simulink model "eCS_Algo_Simulation_2015b_opti - Copy"  (R2015b)
settings: Solver=ode1  StartTime=0.0  StopTime=3  FixedStep=1/80000  RelTol=1e-3
PreLoadFcn:
  | if exist('tl_preloadfcn','file'), tl_preloadfcn(gcs,402); end
PostLoadFcn:
  | , if any(exist('dsrtsu_mdlpostloadfcn', 'file') == [2, 3, 6]), try dsrtsu_mdlpostloadfcn('Execute', bdroot); catch fprintf('Error in PostLoadFcn (dsrtsu_mdlpostloadfcn) for model "%s":\n %s\n', bdroot, lasterr); end, end,
  | if exist('tl_postloadfcn','file'), tl_postloadfcn(gcs,402); end
InitFcn:
  | Omegan=1.3024e+03;
  | xi=0.9; %0.48
  | K=0.1931;
  | K1=0.0198;
  | TauLocked=0.00255;
  | TauUnLocked=0.0042;
  | Kp=1/(2*K1);
  | Ki=Kp/((TauLocked+TauUnLocked)/2);
  | if exist('tlds_init','file'), tlds_init(gcs); end
StartFcn:
  | if exist('tlds_start','file'), tlds_start(gcs); end
StopFcn:
  | if exist('tlds_stop','file'), tlds_stop(gcs); end
model workspace (MAT data in the model file):
  au8PrevExecProfile = [0 0 0 0 0 0]
values from neighbouring files (symbols this model uses):
  AccSensor = 5    [Parameter_eCS_Algo.m]
  AlgoType = 0    [Parameter_eCS_Algo.m]
  Cxy = 1*0.017    (= 0.017)    [Acc_Init_SelV1.m]
  Cxz = 1*0.017    (= 0.017)    [Acc_Init_SelV1.m]
  Cyx = 1*0.017    (= 0.017)    [Acc_Init_SelV1.m]
  Cyz = 1*0.017    (= 0.017)    [Acc_Init_SelV1.m]
  Czx = 1*0.017    (= 0.017)    [Acc_Init_SelV1.m]
  Czy = 1*0.017    (= 0.017)    [Acc_Init_SelV1.m]
  Forced_Oscillation = 0    [Parameter_eCS_Algo.m]    (also in run_Rotation_sim.m = run)
  FreqTemperature = 10    [Acc_Init_SelV1.m]
  MaxSensorOffset = 0.3    [Acc_Init_SelV1.m]
  Mean_x_noise = 4e-3    (= 0.004)    [Acc_Init_SelV1.m]
  Mean_y_noise = 4e-3    (= 0.004)    [Acc_Init_SelV1.m]
  Mean_z_noise = 4e-3    (= 0.004)    [Acc_Init_SelV1.m]
  ODR = 8000    [Acc_Init_SelV1.m]
  offsetcorrection_on_off = 0    [Parameter_eCS_Algo.m]
  phi_pulse_rotation = 0    [Parameter_eCS_Algo.m]    (also in run_Rotation_sim.m = angle)
  pulsetype = 2    [Parameter_eCS_Algo.m]    (also in run_simulation.m = j; run_simulation_ActiveX.m = j)
  Range = 4    [Acc_Init_SelV1.m]
  sensitivity_optimisation = 0    [Parameter_eCS_Algo.m]
  TempBias = 0    [Acc_Init_SelV1.m]
  TemperatureAmp = 0    [Acc_Init_SelV1.m]
  Var_x_noise = 1.84e-9    (= 1.84e-09)    [Acc_Init_SelV1.m]
  Var_y_noise = 2.025e-09    [Acc_Init_SelV1.m]
  Var_z_noise = 1.374e-09    [Acc_Init_SelV1.m]
  w_x = 2*pi*F_x    (= 376.991118431)    [Acc_Init_SelV1.m]
  w_y = 2*pi*F_y    (= 376.991118431)    [Acc_Init_SelV1.m]
  w_z = 2*pi*F_z    (= 376.991118431)    [Acc_Init_SelV1.m]
  x_max_temp_drift = 0.061    [Acc_Init_SelV1.m]
  x_offset_enable = 0    [Acc_Init_SelV1.m]
  x_run_to_run_drift = 0.0    (= 0)    [Acc_Init_SelV1.m]
  x_temp_co_drift = 0.000    (= 0)    [Acc_Init_SelV1.m]
  Xi_x = 0.7    [Acc_Init_SelV1.m]
  Xi_y = 0.7    [Acc_Init_SelV1.m]
  Xi_z = 0.7    [Acc_Init_SelV1.m]
  y_max_temp_drift = 0.061    [Acc_Init_SelV1.m]
  y_offset_enable = 0    [Acc_Init_SelV1.m]
  y_run_to_run_drift = 0.0    (= 0)    [Acc_Init_SelV1.m]
  y_temp_co_drift = 0.000    (= 0)    [Acc_Init_SelV1.m]
  z_max_temp_drift = 0.13    [Acc_Init_SelV1.m]
  z_offset_enable = 0    [Acc_Init_SelV1.m]
  z_run_to_run_drift = 0.0    (= 0)    [Acc_Init_SelV1.m]
  z_temp_co_drift = 0.000    (= 0)    [Acc_Init_SelV1.m]
undefined symbols (not defined in the file or in its folder): ddv, DiscIntNeverNeededParam, gmw_roada_x__m_s__, gmw_roada_y__m_s__, gmw_roadtime_2kHz, KSF_50_a_x, KSF_50_a_y, KSF_50_time, KSG_30_a_x, KSG_30_a_y, KSG_30_time, Meldorf_HindenburgstraAcceleration_x__m_s_2_, Meldorf_HindenburgstraAcceleration_y__m_s_2_, Meldorf_HindenburgstraAcceleration_z__m_s_2_, Meldorf_HindenburgstraTime__s_, pulse_FF27, pulse_MPDB, pulse_ODB40, pulse_ODB64, pulse_USNCAP, pulsetime_FF27, pulsetime_MPDB, pulsetime_ODB40, pulsetime_ODB64, pulsetime_USNCAP, Rauasphalt_60_a_x, Rauasphalt_60_a_y, Rauasphalt_60_time, sigbuilder_block, VW_416_2kHza_x_2kHz, VW_416_2kHza_y_2kHz, VW_416_2kHztime_2kHz
libraries: tllib x22, simulink x20, tl_autosar_lib x10, simulink_extras x7, LIB_TF_G_12_StepControl x2, LIB_TF_G_111 x1, LIB_TF_G_112 x1
(part 2 of 9)

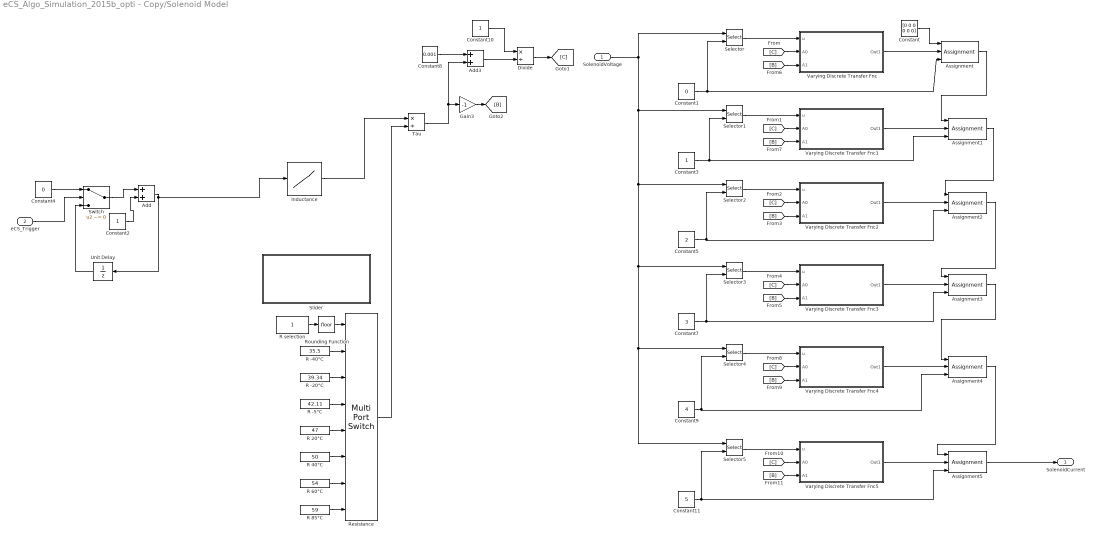
== system eCS_Algo_Simulation_2015b_opti - Copy/Solenoid Model ==
  SolenoidVoltage : Inport
  eCS_Trigger : Inport  Port=2  SampleTime=0.001
  Add : Sum
  Add3 : Sum
  Assignment{,1..5} (6 alike) : Assignment  IndexMode=Zero-based  IndexOptions=Index vector (port)  Indices=1  OutputSizes=1
  Constant : Constant  Value=[0 0 0 0 0 0]
  Constant1 : Constant  Value=0
  Constant10 : Constant
  Constant11 : Constant  Value=5
  Constant2 : Constant
  Constant3 : Constant
  Constant4 : Constant  Value=0
  Constant5 : Constant  Value=2
  Constant7 : Constant  Value=3
  Constant8 : Constant  Value=0.001
  Constant9 : Constant  Value=4
  Divide : Product  Inputs=*/
  Gain3 : Gain  Gain=-1
  Inductance : Lookup_n-D  NumberOfTableDimensions=1  BreakpointsForDimension1=[0 5 10 15 20 25 25.001]  Table=[0.262 0.2108 0.1697 0.1449 0.1286 0.1185 0.1185]  InternalRulePriority=Speed  RndMeth=Simplest  InputSameDT=on
  R -20°C : Constant  Value=39.34
  R -40°C : Constant  Value=35.5
  R -5°C : Constant  Value=42.11
  R 20°C : Constant  Value=47
  R 40°C : Constant  Value=50
  R 60°C : Constant  Value=54
  R 85°C : Constant  Value=59
  R selection : Constant
  Resistance : MultiPortSwitch  Inputs=7
  Rounding Function : Rounding
  Selector{,1..5} (6 alike) : Selector  IndexMode=Zero-based  InputPortWidth=6  IndexOptions=Index vector (port)  Indices=[1 3]  OutputSizes=1
  Slider : Subsystem  DialogController=hmiCreateDDGDialog  IsWebBlock=on  mask(MWDashboardBlock){webBlockId=75143694-038a-4636-9846-8391abf771a2, webBlockType=slider, ShowInLibBrowser=on, ShowInitialText=on, HMISrcModelName=eCS_Algo_Simulation_2015b_opti}
      mask prompts: webBlockId "WebBlock Id"; webBlockType "WebBlock Type"; HMISrcModelName "Source Model"
      mask Help: helpview([docroot '/mapfiles/simulink.map'], 'hmi_slider')
      mask Display:
      | if strcmp(get_param(bdroot(gcb),'BlockDiagramType'), 'library')
      |     image([(matlabroot) '/toolbox/simulink/hmi/icons/Slider.png']);
      | end
  Switch : Switch  Criteria=u2 ~= 0
  Tau : Product  Inputs=*/
  Unit Delay : UnitDelay  SampleTime=-1
  Varying Discrete Transfer Fnc : Subsystem
  Varying Discrete Transfer Fnc1 : Subsystem
  Varying Discrete Transfer Fnc2 : Subsystem
  Varying Discrete Transfer Fnc3 : Subsystem
  Varying Discrete Transfer Fnc4 : Subsystem
  Varying Discrete Transfer Fnc5 : Subsystem
  SolenoidCurrent : Outport
  wires:
  Constant1/1 -> Assignment/3, Selector/2
  Constant/1 -> Assignment/1
  Constant3/1 -> Assignment1/3, Selector1/2
  Assignment/1 -> Assignment1/1
  Constant2/1 -> Add/2
  Add/1 -> Unit Delay/1, Inductance/1
  Switch/1 -> Add/1
  Unit Delay/1 -> Switch/3
  Constant4/1 -> Switch/1
  eCS_Trigger/1 -> Switch/2
  Constant5/1 -> Assignment2/3, Selector2/2
  Assignment1/1 -> Assignment2/1
  Constant7/1 -> Assignment3/3, Selector3/2
  Assignment2/1 -> Assignment3/1
  Constant9/1 -> Assignment4/3, Selector4/2
  Assignment3/1 -> Assignment4/1
  Constant11/1 -> Assignment5/3, Selector5/2
  Assignment4/1 -> Assignment5/1
  SolenoidVoltage/1 -> Selector5/1, Selector4/1, Selector3/1, Selector2/1, Selector1/1, Selector/1
  Assignment5/1 -> SolenoidCurrent/1
  R -40°C/1 -> Resistance/2
  R -20°C/1 -> Resistance/3
  R -5°C/1 -> Resistance/4
  R 20°C/1 -> Resistance/5
  R 40°C/1 -> Resistance/6
  R 60°C/1 -> Resistance/7
  R 85°C/1 -> Resistance/8
  R selection/1 -> Rounding Function/1
  Resistance/1 -> Tau/2
  Tau/1 -> Gain3/1, Add3/2
  Constant8/1 -> Add3/1
  Add3/1 -> Divide/2
  Constant10/1 -> Divide/1
  Divide/1 -> [C]
  Gain3/1 -> [B]
  Rounding Function/1 -> Resistance/1
  Selector/1 -> Varying Discrete Transfer Fnc/1(u)
  Varying Discrete Transfer Fnc/1(Out1) -> Assignment/2
  [C] -> Varying Discrete Transfer Fnc/2(A0)
  [B] -> Varying Discrete Transfer Fnc/3(A1)
  Selector1/1 -> Varying Discrete Transfer Fnc1/1(u)
  [C] -> Varying Discrete Transfer Fnc1/2(A0)
  [B] -> Varying Discrete Transfer Fnc1/3(A1)
  Varying Discrete Transfer Fnc1/1(Out1) -> Assignment1/2
  Selector2/1 -> Varying Discrete Transfer Fnc2/1(u)
  [C] -> Varying Discrete Transfer Fnc2/2(A0)
  [B] -> Varying Discrete Transfer Fnc2/3(A1)
  Varying Discrete Transfer Fnc2/1(Out1) -> Assignment2/2
  Selector3/1 -> Varying Discrete Transfer Fnc3/1(u)
  [C] -> Varying Discrete Transfer Fnc3/2(A0)
  [B] -> Varying Discrete Transfer Fnc3/3(A1)
  Varying Discrete Transfer Fnc3/1(Out1) -> Assignment3/2
  Selector4/1 -> Varying Discrete Transfer Fnc4/1(u)
  [C] -> Varying Discrete Transfer Fnc4/2(A0)
  [B] -> Varying Discrete Transfer Fnc4/3(A1)
  Varying Discrete Transfer Fnc4/1(Out1) -> Assignment4/2
  Selector5/1 -> Varying Discrete Transfer Fnc5/1(u)
  [C] -> Varying Discrete Transfer Fnc5/2(A0)
  [B] -> Varying Discrete Transfer Fnc5/3(A1)
  Varying Discrete Transfer Fnc5/1(Out1) -> Assignment5/2
  Inductance/1 -> Tau/1

== system eCS_Algo_Simulation_2015b_opti - Copy/eCS ==
  prrAccelMtrPerSecSqd : Inport
  prrEcsDiagRequest : Inport  Port=2
  Subsystem : Subsystem  Tag=struct('sfcnName','eCS_sf','subFunction','','srcSubsystem','')  mask(TL_Enable){}
      settings: OpenFcn=warndlg(get_param(gcb,'MaskHelp'),'Serious Warning');
      mask Help: This subsystem keeps the TargetLink subsystem (subsystem with TargetLink blocks for production code generation), and is needed for the TargetLink simulation frame to work properly. DO NOT DELETE OR MODIFY IT!
  psrEcsAlgoData : Outport
  wires:
  prrAccelMtrPerSecSqd/1 -> Subsystem/1(prrAccelMtrPerSecSqd)
  prrEcsDiagRequest/1 -> Subsystem/2(prrEcsDiagRequest)
  Subsystem/1(psrEcsAlgoData) -> psrEcsAlgoData/1

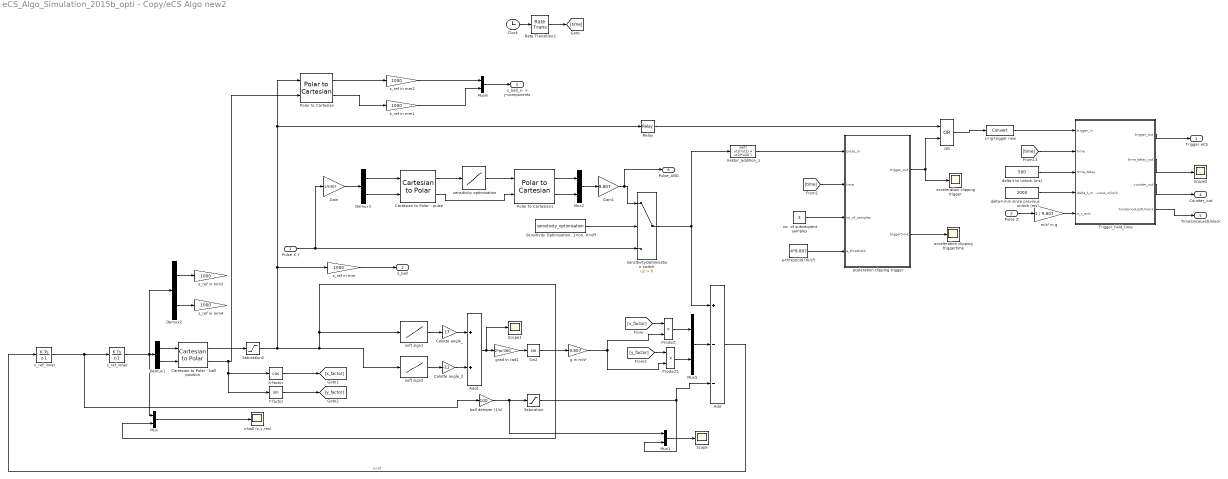
== system eCS_Algo_Simulation_2015b_opti - Copy/eCS Algo new2 ==
  Pulse X,Y : Inport
  Pulse Z : Inport  Port=2
  Add : Sum  Inputs=+--
  Add1 : Sum
  Calotte angle_ : Gain  Gain=17
  Calotte angle_2 : Gain  Gain=-12
  Cartesian to Polar - ball position : simulink_extras/Transformations/Cartesian to Polar
  Cartesian to Polar - pulse : simulink_extras/Transformations/Cartesian to Polar
  Clock : Clock
  Demux1 : Demux  Outputs=2
  Demux2 : Demux  Outputs=2
  Demux3 : Demux  Outputs=2
  Gain : Gain  Gain=1/9.807
  Gain1 : Gain  Gain=9.807
  Mux{,1..2,5..6} (5 alike) : Mux  Inputs=2
  OR : Logic  Operator=OR  AllPortsSameDT=off  OutDataTypeStr=boolean
  Polar to Cartesian : simulink_extras/Transformations/Polar to Cartesian
  Polar to Cartesian1 : simulink_extras/Transformations/Polar to Cartesian
  Product : Product
  Product1 : Product
  Rate Transition2 : RateTransition
  Relay : Relay  OnSwitchValue=0.0004  OffSwitchValue=0.0001
  Saturation : Saturate  UpperLimit=50  LowerLimit=-50
  Saturation2 : Saturate  UpperLimit=0.001  LowerLimit=0
  Scope : Scope
  Scope1 : Scope
  Scope2 : Scope
  "Sensitivity Optimisation: 1=on, 0=off" : Constant  Value=sensitivity_optimisation
  SensitivityOptimisation switch : Switch  Criteria=u2 > Threshold
  Sin2 : Trigonometry
  Trigger_hold_time : MATLAB Function  TreatAsAtomicUnit=on
  Vektor_addition_1 : Fcn  Expr=sqrt( u(1)*u(1) + u(2)*u(2) )
  X-factor : Trigonometry  Operator=cos
  Y-factor : Trigonometry
  a-threshold (m/s²) : Constant  Value=4*9.807
  acceleration clipping trigger : Scope
  acceleration clipping triggertime : Scope
  aceleration clipping trigger : MATLAB Function  TreatAsAtomicUnit=on
  ball damper (1/s) : Gain  Gain=100
  delta-t to unlock (ms) : Constant  Value=500  OutMin=[0]
  delta-t-min since previous unlock (ms) : Constant  Value=2000  OutMin=[0]
  g in m/s² : Gain  Gain=9.807
  grad in rad1 : Gain  Gain=2*pi/360
  m/s² in g : Gain  Gain=1 / 9.807
  no. of subsequent samples : Constant  Value=3
  s-ball (x,y,res) : Scope
  s-rig-trigger new : DataTypeConversion
  s_ref in mm{,1..4} (5 alike) : Gain  Gain=1000
  s_ref_inner : DiscreteIntegrator  InitialConditionSetting=State (most efficient)  SampleTime=-1  LimitOutput=on  UpperSaturationLimit=0.001  LowerSaturationLimit=-0.001  ICPrevOutput=DiscIntNeverNeededParam  ICPrevScaledInput=DiscIntNeverNeededParam
  sensitivity optimisation : Lookup_n-D  NumberOfTableDimensions=1  BreakpointsForDimension1=[0 0.3 0.4 0.5 0.7]  Table=[0 0.2 0.4 0.6 1.2]  UseLastTableValue=on  InternalRulePriority=Speed  RndMeth=Simplest  InputSameDT=on
  soft sign1 : Lookup_n-D  NumberOfTableDimensions=1  BreakpointsForDimension1=[0 0.00002 0.002]  Table=[0 1 1]  ExtrapMethod=Clip  UseLastTableValue=on  InternalRulePriority=Speed  RndMeth=Simplest  InputSameDT=on
  soft sign2 : Lookup_n-D  NumberOfTableDimensions=1  BreakpointsForDimension1="[0 0.0004 0.0005  0.001]"  Table="[0  0 1 1]"  ExtrapMethod=Clip  UseLastTableValue=on  InternalRulePriority=Speed  RndMeth=Simplest  InputSameDT=on
  v_ref_inner : DiscreteIntegrator  InitialConditionSetting=State (most efficient)  SampleTime=-1  ICPrevOutput=DiscIntNeverNeededParam  ICPrevScaledInput=DiscIntNeverNeededParam
  Trigger eCS : Outport
  s_ball : Outport  Port=2
  s_ball_x- + y-components : Outport  Port=3
  Counter_out : Outport  Port=4
  TimeSinceLastUnlock : Outport  Port=5
  Pulse_ANG : Outport  Port=6
  wires:
  v_ref_inner/1 -> s_ref_inner/1, ball damper (1/s)/1
  grad in rad1/1 -> Sin2/1
  soft sign1/1 -> Calotte angle_/1
  Calotte angle_/1 -> Add1/1
  soft sign2/1 -> Calotte angle_2/1
  Calotte angle_2/1 -> Add1/2
  Add1/1 -> Scope1/1, grad in rad1/1
  Sin2/1 -> g in m/s²/1
  Cartesian to Polar - ball position/1 -> Saturation2/1
  ball damper (1/s)/1 -> Mux1/1, Saturation/1
  s_ref in mm/1 -> s_ball/1
  Add/1 -> v_ref_inner/1  "a-ref"
  Mux/1 -> s-ball (x,y,res)/1
  Saturation/1 -> Add/3, Mux1/2
  Mux1/1 -> Scope/1
  Clock/1 -> Rate Transition2/1
  aceleration clipping trigger/2(triggertime) -> acceleration clipping triggertime/1
  no. of subsequent samples/1 -> aceleration clipping trigger/3(no_of_samples)
  a-threshold (m/s²)/1 -> aceleration clipping trigger/4(a_threshold)
  aceleration clipping trigger/1(trigger_out) -> acceleration clipping trigger/1, OR/2
  Relay/1 -> OR/1
  Vektor_addition_1/1 -> aceleration clipping trigger/1(pulse_in)
  [time] -> Trigger_hold_time/2(time)
  Rate Transition2/1 -> [time]
  [time] -> aceleration clipping trigger/2(time)
  delta-t to unlock (ms)/1 -> Trigger_hold_time/3(time_delay)
  OR/1 -> s-rig-trigger new/1
  s-rig-trigger new/1 -> Trigger_hold_time/1(trigger_in)
  delta-t-min since previous unlock (ms)/1 -> Trigger_hold_time/4(delta_t_min_since_previous_unlock)
  Trigger_hold_time/1(trigger_out) -> Trigger eCS/1
  Trigger_hold_time/2(time_delay_out) -> Scope2/1
  Demux1/2 -> Cartesian to Polar - ball position/2
  Demux1/1 -> Cartesian to Polar - ball position/1
  s_ref_inner/1 -> Demux2/1, Mux/1, Demux1/1
  Cartesian to Polar - ball position/2 -> Polar to Cartesian/2, Y-factor/1, X-factor/1
  Mux5/1 -> Add/2
  Product/1 -> Mux5/1
  Product1/1 -> Mux5/2
  g in m/s²/1 -> Product1/2, Product/2
  [x_factor] -> Product/1
  [y_factor] -> Product1/1
  X-factor/1 -> [x_factor]
  Y-factor/1 -> [y_factor]
  Saturation2/1 -> soft sign2/1, soft sign1/1, Mux/2, Polar to Cartesian/1, Relay/1, s_ref in mm/1
  Demux2/1 -> s_ref in mm3/1
  Demux2/2 -> s_ref in mm4/1
  Polar to Cartesian/2 -> s_ref in mm1/1
  Polar to Cartesian/1 -> s_ref in mm2/1
  Mux6/1 -> s_ball_x- + y-components/1
  s_ref in mm1/1 -> Mux6/2
  s_ref in mm2/1 -> Mux6/1
  Pulse Z/1 -> m/s² in g/1
  m/s² in g/1 -> Trigger_hold_time/5(a_z_axis)
  Trigger_hold_time/3(counter_out) -> Counter_out/1
  Trigger_hold_time/4(timeSinceLastUnlock) -> TimeSinceLastUnlock/1
  SensitivityOptimisation switch/1 -> Add/1, Vektor_addition_1/1
  Pulse X,Y/1 -> Gain/1, SensitivityOptimisation switch/3
  Gain1/1 -> Pulse_ANG/1, SensitivityOptimisation switch/1
  "Sensitivity Optimisation: 1=on, 0=off"/1 -> SensitivityOptimisation switch/2
  Demux3/1 -> Cartesian to Polar - pulse/1
  Demux3/2 -> Cartesian to Polar - pulse/2
  sensitivity optimisation/1 -> Polar to Cartesian1/1
  Cartesian to Polar - pulse/2 -> Polar to Cartesian1/2
  Cartesian to Polar - pulse/1 -> sensitivity optimisation/1
  Polar to Cartesian1/2 -> Mux2/2
  Polar to Cartesian1/1 -> Mux2/1
  Mux2/1 -> Gain1/1
  Gain/1 -> Demux3/1

== system eCS_Algo_Simulation_2015b_opti - Copy/eCS_prrEcsDiagRequest_b8DiagReq1 ==
  Const : Constant  Value=85
  b8DiagReq : Outport
  wires:
  Const/1 -> b8DiagReq/1  "b8DiagReq"

== system eCS_Algo_Simulation_2015b_opti - Copy/oscilliation generator ==
  bOscillationReq : Inport
  Constant1 : Constant  Value=0
  Constant3 : Constant  Value=0
  Constant5 : Constant  Value=0
  Sine Wave : Sin  Amplitude=0.2  Frequency=6280  Phase=3.14/2  SampleTime=0
  Sine Wave2 : Sin  Amplitude=0.2  Frequency=1256  SampleTime=0
  Switch1 : Switch  Criteria=u2 ~= 0
  Switch2 : Switch  Criteria=u2 ~= 0
  Switch3 : Switch  Criteria=u2 ~= 0
  Oscillation_ax : Outport
  Oscillation_ay : Outport  Port=2
  Oscillation_az : Outport  Port=3
  wires:
  Switch1/1 -> Oscillation_ax/1
  Sine Wave/1 -> Switch2/1, Switch1/1
  Constant3/1 -> Switch1/3
  Constant5/1 -> Switch2/3
  Switch2/1 -> Oscillation_ay/1
  Sine Wave2/1 -> Switch3/1
  Constant1/1 -> Switch3/3
  bOscillationReq/1 -> Switch3/2, Switch2/2, Switch1/2
  Switch3/1 -> Oscillation_az/1

== system eCS_Algo_Simulation_2015b_opti - Copy/pulse rotation around z-axis ==
  pulse in m/s² : Inport
  rotation angle : Inport  Port=2
  Enable : EnablePort
  Add5 : Sum
  Cartesian to Polar : simulink_extras/Transformations/Cartesian to Polar
  Degrees to Radians : simulink_extras/Transformations/Degrees to Radians
  Demux1 : Demux  Outputs=2
  Mux10 : Mux  Inputs=2
  Polar to Cartesian : simulink_extras/Transformations/Polar to Cartesian
  pulse rotated in m/s² : Outport
  wires:
  rotation angle/1 -> Degrees to Radians/1
  Degrees to Radians/1 -> Add5/2
  Demux1/2 -> Cartesian to Polar/2
  Add5/1 -> Polar to Cartesian/2
  Cartesian to Polar/1 -> Polar to Cartesian/1
  Demux1/1 -> Cartesian to Polar/1
  Cartesian to Polar/2 -> Add5/1
  Polar to Cartesian/1 -> Mux10/1
  Polar to Cartesian/2 -> Mux10/2
  pulse in m/s²/1 -> Demux1/1
  Mux10/1 -> pulse rotated in m/s²/1  "pulse rotated in m/s²"

== system eCS_Algo_Simulation_2015b_opti - Copy/FSM/Subsystem ==
  prrEcsAlgoFlag : Inport
  prrVehicleInputs : Inport  Port=2
  FSM : Subsystem  Tag=MIL Subsystem  Description=b  mask(MIL Subsystem){}
      settings: CopyFcn=if exist('tl_copyfcn','file'), tl_copyfcn(gcbh); end  NameChangeFcn=if exist('tl_namechangefcn','file'), tl_namechangefcn(gcbh); end  DestroyFcn=if exist('update_tl_main_dlg','file'), update_tl_main_dlg('TL_subs_display'); end
  psrSolenoidState : Outport
  psrFsmProfile : Outport  Port=2
  wires:
  prrEcsAlgoFlag/1 -> FSM/1(prrEcsAlgoFlag)
  prrVehicleInputs/1 -> FSM/2(prrVehicleInputs)
  FSM/1(psrSolenoidState) -> psrSolenoidState/1
  FSM/2(psrFsmProfile) -> psrFsmProfile/1

== system eCS_Algo_Simulation_2015b_opti - Copy/Input (Pulse// Angle)1/Puls_BMW_KSF_50 ==
  time in : Inport
  Constant : Constant  Value=KSF_50_time
  Constant1 : Constant  Value=KSF_50_a_x
  Constant3 : Constant  Value=KSF_50_a_y
  Lookup Table Dynamic : simulink/Lookup Tables/Lookup Table Dynamic  LookUpMeth=Interpolation-Use End Values  OutDataTypeStr=fixdt('double')  OutputDataTypeScalingMode=Specify via dialog  OutDataType=fixdt('double')  OutScaling=[]  DoSatur=off
  Lookup Table Dynamic1 : simulink/Lookup Tables/Lookup Table Dynamic  LookUpMeth=Interpolation-Use End Values  OutDataTypeStr=fixdt('double')  OutputDataTypeScalingMode=Specify via dialog  OutDataType=fixdt('double')  OutScaling=[]  DoSatur=off
  Mux : Mux  Inputs=2
  Rate Transition1 : RateTransition
  Rate Transition2 : RateTransition  OutPortSampleTime=1/2000
  Scope : Scope
  m/s² to g : Gain  Gain=1/9.81
  pulse out [x,y] (g) : Outport
  wires:
  Lookup Table Dynamic/1 -> Mux/1
  Rate Transition2/1 -> Lookup Table Dynamic1/1, Lookup Table Dynamic/1
  Lookup Table Dynamic1/1 -> Mux/2
  time in/1 -> Rate Transition2/1
  Constant1/1 -> Lookup Table Dynamic/3
  Constant/1 -> Lookup Table Dynamic1/2, Lookup Table Dynamic/2
  Constant3/1 -> Lookup Table Dynamic1/3
  Rate Transition1/1 -> Scope/1, pulse out [x,y] (g)/1
  m/s² to g/1 -> Rate Transition1/1
  Mux/1 -> m/s² to g/1

== system eCS_Algo_Simulation_2015b_opti - Copy/Input (Pulse// Angle)1/Puls_BMW_KSG_30 ==
  time in : Inport
  Constant : Constant  Value=KSG_30_time
  Constant1 : Constant  Value=KSG_30_a_x
  Constant3 : Constant  Value=KSG_30_a_y
  Lookup Table Dynamic : simulink/Lookup Tables/Lookup Table Dynamic  LookUpMeth=Interpolation-Use End Values  OutDataTypeStr=fixdt('double')  OutputDataTypeScalingMode=Specify via dialog  OutDataType=fixdt('double')  OutScaling=[]  DoSatur=off
  Lookup Table Dynamic1 : simulink/Lookup Tables/Lookup Table Dynamic  LookUpMeth=Interpolation-Use End Values  OutDataTypeStr=fixdt('double')  OutputDataTypeScalingMode=Specify via dialog  OutDataType=fixdt('double')  OutScaling=[]  DoSatur=off
  Mux : Mux  Inputs=2
  Rate Transition1 : RateTransition
  Rate Transition2 : RateTransition  OutPortSampleTime=1/2000
  Scope : Scope
  m/s² to g : Gain  Gain=1/9.81
  pulse out [x,y] (g) : Outport
  wires:
  Mux/1 -> m/s² to g/1
  m/s² to g/1 -> Rate Transition1/1
  Rate Transition1/1 -> pulse out [x,y] (g)/1, Scope/1
  Constant3/1 -> Lookup Table Dynamic1/3
  Constant/1 -> Lookup Table Dynamic/2, Lookup Table Dynamic1/2
  Constant1/1 -> Lookup Table Dynamic/3
  time in/1 -> Rate Transition2/1
  Lookup Table Dynamic1/1 -> Mux/2
  Rate Transition2/1 -> Lookup Table Dynamic/1, Lookup Table Dynamic1/1
  Lookup Table Dynamic/1 -> Mux/1

== system eCS_Algo_Simulation_2015b_opti - Copy/Input (Pulse// Angle)1/Puls_BMW_Rauasphalt_60  ==
  time in : Inport
  Constant : Constant  Value=Rauasphalt_60_time
  Constant1 : Constant  Value=Rauasphalt_60_a_x
  Constant3 : Constant  Value=Rauasphalt_60_a_y
  Lookup Table Dynamic : simulink/Lookup Tables/Lookup Table Dynamic  LookUpMeth=Interpolation-Use End Values  OutDataTypeStr=fixdt('double')  OutputDataTypeScalingMode=Specify via dialog  OutDataType=fixdt('double')  OutScaling=[]  DoSatur=off
  Lookup Table Dynamic1 : simulink/Lookup Tables/Lookup Table Dynamic  LookUpMeth=Interpolation-Use End Values  OutDataTypeStr=fixdt('double')  OutputDataTypeScalingMode=Specify via dialog  OutDataType=fixdt('double')  OutScaling=[]  DoSatur=off
  Mux : Mux  Inputs=2
  Rate Transition1 : RateTransition
  Rate Transition2 : RateTransition  OutPortSampleTime=1/2000
  Scope : Scope
  m/s² to g : Gain  Gain=1/9.81
  pulse out [x,y] (g) : Outport
  wires:
  Lookup Table Dynamic/1 -> Mux/1
  Rate Transition2/1 -> Lookup Table Dynamic1/1, Lookup Table Dynamic/1
  Lookup Table Dynamic1/1 -> Mux/2
  time in/1 -> Rate Transition2/1
  Constant1/1 -> Lookup Table Dynamic/3
  Constant/1 -> Lookup Table Dynamic1/2, Lookup Table Dynamic/2
  Constant3/1 -> Lookup Table Dynamic1/3
  Rate Transition1/1 -> Scope/1, pulse out [x,y] (g)/1
  m/s² to g/1 -> Rate Transition1/1
  Mux/1 -> m/s² to g/1

== system eCS_Algo_Simulation_2015b_opti - Copy/Input (Pulse// Angle)1/Puls_GWM_road_C.Morgan ==
  time in : Inport
  Constant : Constant  Value=gmw_roadtime_2kHz
  Constant1 : Constant  Value=gmw_roada_x__m_s__
  Constant3 : Constant  Value=gmw_roada_y__m_s__
  Lookup Table Dynamic : simulink/Lookup Tables/Lookup Table Dynamic  LookUpMeth=Interpolation-Use End Values  OutDataTypeStr=fixdt('double')  OutputDataTypeScalingMode=Specify via dialog  OutDataType=fixdt('double')  OutScaling=[]  DoSatur=off
  Lookup Table Dynamic1 : simulink/Lookup Tables/Lookup Table Dynamic  LookUpMeth=Interpolation-Use End Values  OutDataTypeStr=fixdt('double')  OutputDataTypeScalingMode=Specify via dialog  OutDataType=fixdt('double')  OutScaling=[]  DoSatur=off
  Mux : Mux  Inputs=2
  Rate Transition1 : RateTransition
  Rate Transition2 : RateTransition  OutPortSampleTime=1/2000
  Scope : Scope
  m/s² to g : Gain  Gain=1/9.81
  pulse out [x,y] (g) : Outport
  wires:
  Mux/1 -> m/s² to g/1
  m/s² to g/1 -> Rate Transition1/1
  Rate Transition1/1 -> pulse out [x,y] (g)/1, Scope/1
  Constant3/1 -> Lookup Table Dynamic1/3
  Constant/1 -> Lookup Table Dynamic/2, Lookup Table Dynamic1/2
  Constant1/1 -> Lookup Table Dynamic/3
  time in/1 -> Rate Transition2/1
  Lookup Table Dynamic1/1 -> Mux/2
  Rate Transition2/1 -> Lookup Table Dynamic/1, Lookup Table Dynamic1/1
  Lookup Table Dynamic/1 -> Mux/1

== system eCS_Algo_Simulation_2015b_opti - Copy/Input (Pulse// Angle)1/Puls_Kopfsteinpflaster Meldorf Hindenburgstrasse ==
  time in : Inport
  Constant : Constant  Value=Meldorf_HindenburgstraTime__s_
  Constant1 : Constant  Value=Meldorf_HindenburgstraAcceleration_x__m_s_2_
  Constant2 : Constant  Value=Meldorf_HindenburgstraAcceleration_z__m_s_2_
  Constant3 : Constant  Value=Meldorf_HindenburgstraAcceleration_y__m_s_2_
  Gain : Gain  Gain=-1
  Lookup Table Dynamic : simulink/Lookup Tables/Lookup Table Dynamic  LookUpMeth=Interpolation-Use End Values  OutDataTypeStr=fixdt('double')  OutputDataTypeScalingMode=Specify via dialog  OutDataType=fixdt('double')  OutScaling=[]  DoSatur=off
  Lookup Table Dynamic1 : simulink/Lookup Tables/Lookup Table Dynamic  LookUpMeth=Interpolation-Use End Values  OutDataTypeStr=fixdt('double')  OutputDataTypeScalingMode=Specify via dialog  OutDataType=fixdt('double')  OutScaling=[]  DoSatur=off
  Lookup Table Dynamic2 : simulink/Lookup Tables/Lookup Table Dynamic  LookUpMeth=Interpolation-Use End Values  OutDataTypeStr=fixdt('double')  OutputDataTypeScalingMode=Specify via dialog  OutDataType=fixdt('double')  OutScaling=[]  DoSatur=off
  Mux : Mux  Inputs=3
  Rate Transition1 : RateTransition
  Rate Transition2 : RateTransition  OutPortSampleTime=1/500
  Scope : Scope
  m/s² to g : Gain  Gain=1/9.81
  pulse out [x,y] (g) : Outport
  wires:
  Lookup Table Dynamic/1 -> Mux/1
  Rate Transition2/1 -> Lookup Table Dynamic2/1, Lookup Table Dynamic1/1, Lookup Table Dynamic/1
  Lookup Table Dynamic1/1 -> Mux/2
  time in/1 -> Rate Transition2/1
  Constant1/1 -> Lookup Table Dynamic/3
  Constant/1 -> Lookup Table Dynamic2/2, Lookup Table Dynamic1/2, Lookup Table Dynamic/2
  Constant3/1 -> Lookup Table Dynamic1/3
  Rate Transition1/1 -> Scope/1, pulse out [x,y] (g)/1
  m/s² to g/1 -> Rate Transition1/1
  Mux/1 -> m/s² to g/1
  Constant2/1 -> Lookup Table Dynamic2/3
  Lookup Table Dynamic2/1 -> Gain/1
  Gain/1 -> Mux/3

== system eCS_Algo_Simulation_2015b_opti - Copy/Input (Pulse// Angle)1/Puls_VW416_Atlas_C.Morgan ==
  time in : Inport
  Constant : Constant  Value=VW_416_2kHztime_2kHz
  Constant1 : Constant  Value=VW_416_2kHza_x_2kHz
  Constant3 : Constant  Value=VW_416_2kHza_y_2kHz
  Lookup Table Dynamic : simulink/Lookup Tables/Lookup Table Dynamic  LookUpMeth=Interpolation-Use End Values  OutDataTypeStr=fixdt('double')  OutputDataTypeScalingMode=Specify via dialog  OutDataType=fixdt('double')  OutScaling=[]  DoSatur=off
  Lookup Table Dynamic1 : simulink/Lookup Tables/Lookup Table Dynamic  LookUpMeth=Interpolation-Use End Values  OutDataTypeStr=fixdt('double')  OutputDataTypeScalingMode=Specify via dialog  OutDataType=fixdt('double')  OutScaling=[]  DoSatur=off
  Mux : Mux  Inputs=2
  Rate Transition1 : RateTransition
  Rate Transition2 : RateTransition  OutPortSampleTime=1/2000
  Scope : Scope
  pulse out [x,y] (g) : Outport
  wires:
  Mux/1 -> Rate Transition1/1
  Rate Transition1/1 -> pulse out [x,y] (g)/1, Scope/1
  Constant3/1 -> Lookup Table Dynamic1/3
  Constant/1 -> Lookup Table Dynamic/2, Lookup Table Dynamic1/2
  Constant1/1 -> Lookup Table Dynamic/3
  time in/1 -> Rate Transition2/1
  Lookup Table Dynamic1/1 -> Mux/2
  Rate Transition2/1 -> Lookup Table Dynamic/1, Lookup Table Dynamic1/1
  Lookup Table Dynamic/1 -> Mux/1

== system eCS_Algo_Simulation_2015b_opti - Copy/SAD/Subsystem ==
  prrFsmProfile : Inport
  sim_au16Current : Inport  Port=2
  SAD : Subsystem  Tag=MIL Subsystem  Description=c  mask(MIL Subsystem){}
      settings: CopyFcn=if exist('tl_copyfcn','file'), tl_copyfcn(gcbh); end  NameChangeFcn=if exist('tl_namechangefcn','file'), tl_namechangefcn(gcbh); end  DestroyFcn=if exist('update_tl_main_dlg','file'), update_tl_main_dlg('TL_subs_display'); end
  pseSolenoidPWM : Outport
  wires:
  prrFsmProfile/1 -> SAD/1(prrFsmProfile)
  sim_au16Current/1 -> SAD/2(sim_au16Current)
  SAD/1(pseSolenoidPWM) -> pseSolenoidPWM/1

== system eCS_Algo_Simulation_2015b_opti - Copy/Solenoid Model/Slider ==

== system eCS_Algo_Simulation_2015b_opti - Copy/Solenoid Model/Varying Discrete Transfer Fnc ==
  u : Inport
  A0 : Inport  Port=2
  A1 : Inport  Port=3
  Add2 : Sum  Inputs=+-
  Gain5 : Gain  Gain=K1*0.001
  Product : Product
  Product1 : Product
  Unit Delay2 : UnitDelay  SampleTime=-1
  Out1 : Outport
  wires:
  Add2/1 -> Product/1
  Product1/1 -> Add2/2
  Product/1 -> Unit Delay2/1
  u/1 -> Add2/1
  Unit Delay2/1 -> Gain5/1, Product1/1
  A0/1 -> Product/2
  A1/1 -> Product1/2
  Gain5/1 -> Out1/1

== system eCS_Algo_Simulation_2015b_opti - Copy/Solenoid Model/Varying Discrete Transfer Fnc1 ==
  u : Inport
  A0 : Inport  Port=2
  A1 : Inport  Port=3
  Add2 : Sum  Inputs=+-
  Gain5 : Gain  Gain=K1*0.001
  Product : Product
  Product1 : Product
  Saturation2 : Saturate  UpperLimit=1  LowerLimit=0
  Unit Delay2 : UnitDelay  SampleTime=-1
  Out1 : Outport
  wires:
  A1/1 -> Product1/2
  A0/1 -> Product/2
  Gain5/1 -> Saturation2/1
  Unit Delay2/1 -> Product1/1, Gain5/1
  u/1 -> Add2/1
  Product/1 -> Unit Delay2/1
  Product1/1 -> Add2/2
  Add2/1 -> Product/1
  Saturation2/1 -> Out1/1

== system eCS_Algo_Simulation_2015b_opti - Copy/Solenoid Model/Varying Discrete Transfer Fnc2 ==
  u : Inport
  A0 : Inport  Port=2
  A1 : Inport  Port=3
  Add2 : Sum  Inputs=+-
  Gain5 : Gain  Gain=K1*0.001
  Product : Product
  Product1 : Product
  Saturation2 : Saturate  UpperLimit=1  LowerLimit=0
  Unit Delay2 : UnitDelay  SampleTime=-1
  Out1 : Outport
  wires:
  Add2/1 -> Product/1
  Product1/1 -> Add2/2
  Product/1 -> Unit Delay2/1
  u/1 -> Add2/1
  Unit Delay2/1 -> Gain5/1, Product1/1
  Gain5/1 -> Saturation2/1
  A0/1 -> Product/2
  A1/1 -> Product1/2
  Saturation2/1 -> Out1/1

== system eCS_Algo_Simulation_2015b_opti - Copy/Solenoid Model/Varying Discrete Transfer Fnc3 ==
  u : Inport
  A0 : Inport  Port=2
  A1 : Inport  Port=3
  Add2 : Sum  Inputs=+-
  Gain5 : Gain  Gain=K1*0.001
  Product : Product
  Product1 : Product
  Saturation2 : Saturate  UpperLimit=1  LowerLimit=0
  Unit Delay2 : UnitDelay  SampleTime=-1
  Out1 : Outport
  wires:
  A1/1 -> Product1/2
  A0/1 -> Product/2
  Gain5/1 -> Saturation2/1
  Unit Delay2/1 -> Product1/1, Gain5/1
  u/1 -> Add2/1
  Product/1 -> Unit Delay2/1
  Product1/1 -> Add2/2
  Add2/1 -> Product/1
  Saturation2/1 -> Out1/1

== system eCS_Algo_Simulation_2015b_opti - Copy/Solenoid Model/Varying Discrete Transfer Fnc4 ==
  u : Inport
  A0 : Inport  Port=2
  A1 : Inport  Port=3
  Add2 : Sum  Inputs=+-
  Gain5 : Gain  Gain=K1*0.001
  Product : Product
  Product1 : Product
  Saturation2 : Saturate  UpperLimit=1  LowerLimit=0
  Unit Delay2 : UnitDelay  SampleTime=-1
  Out1 : Outport
  wires:
  Add2/1 -> Product/1
  Product1/1 -> Add2/2
  Product/1 -> Unit Delay2/1
  u/1 -> Add2/1
  Unit Delay2/1 -> Gain5/1, Product1/1
  Gain5/1 -> Saturation2/1
  A0/1 -> Product/2
  A1/1 -> Product1/2
  Saturation2/1 -> Out1/1

== system eCS_Algo_Simulation_2015b_opti - Copy/Solenoid Model/Varying Discrete Transfer Fnc5 ==
  u : Inport
  A0 : Inport  Port=2
  A1 : Inport  Port=3
  Add2 : Sum  Inputs=+-
  Gain5 : Gain  Gain=K1*0.001
  Product : Product
  Product1 : Product
  Saturation2 : Saturate  UpperLimit=1  LowerLimit=0
  Unit Delay2 : UnitDelay  SampleTime=-1
  Out1 : Outport
  wires:
  A1/1 -> Product1/2
  A0/1 -> Product/2
  Gain5/1 -> Saturation2/1
  Unit Delay2/1 -> Product1/1, Gain5/1
  u/1 -> Add2/1
  Product/1 -> Unit Delay2/1
  Product1/1 -> Add2/2
  Add2/1 -> Product/1
  Saturation2/1 -> Out1/1

== system eCS_Algo_Simulation_2015b_opti - Copy/eCS/Subsystem ==
  prrAccelMtrPerSecSqd : Inport
  prrEcsDiagRequest : Inport  Port=2
  eCS : Subsystem  Tag=MIL Subsystem  Description=d  mask(MIL Subsystem){}
      settings: CopyFcn=if exist('tl_copyfcn','file'), tl_copyfcn(gcbh); end  NameChangeFcn=if exist('tl_namechangefcn','file'), tl_namechangefcn(gcbh); end  DestroyFcn=if exist('update_tl_main_dlg','file'), update_tl_main_dlg('TL_subs_display'); end
  psrEcsAlgoData : Outport
  wires:
  prrAccelMtrPerSecSqd/1 -> eCS/1(prrAccelMtrPerSecSqd)
  prrEcsDiagRequest/1 -> eCS/2(prrEcsDiagRequest)
  eCS/1(psrEcsAlgoData) -> psrEcsAlgoData/1

== system eCS_Algo_Simulation_2015b_opti - Copy/FSM/Subsystem/FSM ==
  prrEcsAlgoFlag : Inport
      settings: NameChangeFcn=if exist('tl_check_ports','file'), tl_check_ports(gcbh); end
      settings: CopyFcn=|
      | if exist('tl_reset_reviewflag','file')==2
      |     tl_reset_reviewflag(gcbh);
      | end
      | if exist('tl_check_ports','file')
      |     tl_check_ports(gcbh);
      | end
  prrVehicleInputs : Inport  Port=2
      settings: NameChangeFcn=if exist('tl_check_ports','file'), tl_check_ports(gcbh); end
      settings: CopyFcn=|
      | if exist('tl_reset_reviewflag','file')==2
      |     tl_reset_reviewflag(gcbh);
      | end
      | if exist('tl_check_ports','file')
      |     tl_check_ports(gcbh);
      | end
  FSM : Subsystem
  psrSolenoidState : Outport
      settings: NameChangeFcn=if exist('tl_check_ports','file'), tl_check_ports(gcbh); end
      settings: CopyFcn=|
      | if exist('tl_reset_reviewflag','file')==2
      |     tl_reset_reviewflag(gcbh);
      | end
      | if exist('tl_check_ports','file')
      |     tl_check_ports(gcbh);
      | end
  psrFsmProfile : Outport  Port=2
      settings: NameChangeFcn=if exist('tl_check_ports','file'), tl_check_ports(gcbh); end
      settings: CopyFcn=|
      | if exist('tl_reset_reviewflag','file')==2
      |     tl_reset_reviewflag(gcbh);
      | end
      | if exist('tl_check_ports','file')
      |     tl_check_ports(gcbh);
      | end
  wires:
  prrEcsAlgoFlag/1 -> FSM/1(prrEcsAlgoFlag)
  prrVehicleInputs/1 -> FSM/2(prrVehicleInputs)
  FSM/1(psrSolenoidState) -> psrSolenoidState/1
  FSM/2(psrFsmProfile) -> psrFsmProfile/1

== system eCS_Algo_Simulation_2015b_opti - Copy/SAD/Subsystem/SAD ==
  prrFsmProfile : Inport
      settings: NameChangeFcn=if exist('tl_check_ports','file'), tl_check_ports(gcbh); end
      settings: CopyFcn=|
      | if exist('tl_reset_reviewflag','file')==2
      |     tl_reset_reviewflag(gcbh);
      | end
      | if exist('tl_check_ports','file')
      |     tl_check_ports(gcbh);
      | end
  sim_au16Current : Inport  Port=2
      settings: NameChangeFcn=if exist('tl_check_ports','file'), tl_check_ports(gcbh); end
      settings: CopyFcn=|
      | if exist('tl_reset_reviewflag','file')==2
      |     tl_reset_reviewflag(gcbh);
      | end
      | if exist('tl_check_ports','file')
      |     tl_check_ports(gcbh);
      | end
  SAD : Subsystem
  pseSolenoidPWM : Outport
      settings: NameChangeFcn=if exist('tl_check_ports','file'), tl_check_ports(gcbh); end
      settings: CopyFcn=|
      | if exist('tl_reset_reviewflag','file')==2
      |     tl_reset_reviewflag(gcbh);
      | end
      | if exist('tl_check_ports','file')
      |     tl_check_ports(gcbh);
      | end
  wires:
  prrFsmProfile/1 -> SAD/1(prrFsmProfile)
  sim_au16Current/1 -> SAD/2(sim_au16Current)
  SAD/1(pseSolenoidPWM) -> pseSolenoidPWM/1

== system eCS_Algo_Simulation_2015b_opti - Copy/eCS/Subsystem/eCS ==
  prrAccelMtrPerSecSqd : Inport
      settings: NameChangeFcn=if exist('tl_check_ports','file'), tl_check_ports(gcbh); end
      settings: CopyFcn=|
      | if exist('tl_reset_reviewflag','file')==2
      |     tl_reset_reviewflag(gcbh);
      | end
      | if exist('tl_check_ports','file')
      |     tl_check_ports(gcbh);
      | end
  prrEcsDiagRequest : Inport  Port=2
      settings: NameChangeFcn=if exist('tl_check_ports','file'), tl_check_ports(gcbh); end
      settings: CopyFcn=|
      | if exist('tl_reset_reviewflag','file')==2
      |     tl_reset_reviewflag(gcbh);
      | end
      | if exist('tl_check_ports','file')
      |     tl_check_ports(gcbh);
      | end
  eCS : Subsystem
  psrEcsAlgoData : Outport
      settings: NameChangeFcn=if exist('tl_check_ports','file'), tl_check_ports(gcbh); end
      settings: CopyFcn=|
      | if exist('tl_reset_reviewflag','file')==2
      |     tl_reset_reviewflag(gcbh);
      | end
      | if exist('tl_check_ports','file')
      |     tl_check_ports(gcbh);
      | end
  wires:
  prrAccelMtrPerSecSqd/1 -> eCS/1(prrAccelMtrPerSecSqd)
  prrEcsDiagRequest/1 -> eCS/2(prrEcsDiagRequest)
  eCS/1(psrEcsAlgoData) -> psrEcsAlgoData/1

== system eCS_Algo_Simulation_2015b_opti - Copy/FSM/Subsystem/FSM/FSM ==
  prrEcsAlgoFlag : Inport
  prrVehicleInputs : Inport  Port=2
  BusSelector : BusSelector  OutputSignals=b8EcsFlag,u16BallPosition
  BusSelector1 : BusSelector  OutputSignals=u16Vx,u8BuckleState
  Constant1 : Constant  Value=ddv('Common/KU8_ONE')  mask(TL_Constant){data={'output',{'variable','Common/KU8_ONE'},'date',738776.66346280091}}
      settings: CopyFcn=if exist('tl_reset_reviewflag','file')==2,tl_reset_reviewflag(gcbh);end  DeleteFcn=if exist('delete_tlblock','file')==2,delete_tlblock(gcbh);end  NameChangeFcn=if exist('rename_tlblock','file')==2,rename_tlblock(gcbh);end  OpenFcn=if exist('tl_open_blockdlg','file')==2,tl_open_blockdlg(gcbh);else,open_system(gcbh,'parameter');end
      mask Help: eval(['if exist(''tl_online_help'',''file'') == 2, tl_online_help(''Topic'',''TL_Constant''),else, web([''jar:file:///'',matlabroot,''/help/toolbox/simulink/help.jar!/slref/' lower(get_param(gcbh,'Blocktype')) '.html''], ''-helpbrowser''),end'])
      mask Display: plot([-0.1, 1.05, NaN, -0.1, 1.05],[.01, .01, NaN, .99, .99]);
  FSM_runCheckModeStatus : Subsystem  TreatAsAtomicUnit=on
  FSM_runCheckVehicleInputs : Subsystem  TreatAsAtomicUnit=on
  FSM_runMainFunction : Subsystem  TreatAsAtomicUnit=on
  PP_psrFsmProfile : tl_autosar_lib/SWC SenderPort  data={'softwarecomponent','AUTOLIV/SoftwareComponents/FSM/FSM','port','psrSolenoidProfile','date',738785.57687237265}  displaystring=FSM\npsrSolenoidProfile
  PP_psrSolenoidState : tl_autosar_lib/SWC SenderPort  data={'softwarecomponent','AUTOLIV/SoftwareComponents/FSM/FSM','port','psrSolenoidState','date',738308.6646808217}  displaystring=FSM\npsrSolenoidState
  RP_prrEcsAlgoFlag : tl_autosar_lib/SWC ReceiverPort  data={'softwarecomponent','AUTOLIV/SoftwareComponents/FSM/FSM','port','prrEcsAlgoFlag','date',738304.65103918978}  displaystring=FSM\nprrEcsAlgoFlag
  RP_prrVehicleInputs : tl_autosar_lib/SWC ReceiverPort  data={'softwarecomponent','AUTOLIV/SoftwareComponents/FSM/FSM','port','prrVehicleInputs','date',738304.65103979164}  displaystring=FSM\nprrVehicleInputs
  Terminator2 : Terminator
  psrSolenoidState : Outport
  psrFsmProfile : Outport  Port=2
  wires:
  prrEcsAlgoFlag/1 -> RP_prrEcsAlgoFlag/1
  RP_prrEcsAlgoFlag/1 -> BusSelector/1
  prrVehicleInputs/1 -> RP_prrVehicleInputs/1
  RP_prrVehicleInputs/1 -> BusSelector1/1
  BusSelector/1 -> FSM_runMainFunction/1(drparg_b8EcsFlag)  "<b8EcsFlag>"
  BusSelector1/1 -> FSM_runCheckVehicleInputs/2(drparg_u16Vx)  "<u16Vx>"
  FSM_runCheckVehicleInputs/1(ab8IsSolenoidUsed) -> FSM_runMainFunction/3(ab8IsSolenoidUsed)  "ab8IsSolenoidUsed"
  PP_psrSolenoidState/1 -> psrSolenoidState/1
  PP_psrFsmProfile/1 -> psrFsmProfile/1
  FSM_runMainFunction/1(au8FsmState) -> PP_psrSolenoidState/1  "au8SolenoidState"
  FSM_runMainFunction/2(au8SelectedProfile) -> PP_psrFsmProfile/1  "au8SelectedProfile"
  BusSelector/2 -> Terminator2/1  "<u16BallPosition>"
  Constant1/1 -> FSM_runCheckModeStatus/1(u32ModesToCheck)
  BusSelector1/2 -> FSM_runCheckVehicleInputs/3(drparg_u8BuckleState)  "<u8BuckleState>"
  FSM_runCheckModeStatus/1(bModeStatus) -> FSM_runCheckVehicleInputs/1(bModeStatus), FSM_runMainFunction/2(bModeStatus)

== system eCS_Algo_Simulation_2015b_opti - Copy/SAD/Subsystem/SAD/SAD ==
  prrFsmProfile : Inport
  sim_au16Current : Inport  Port=2
  PP_pseSolenoidPWM : tl_autosar_lib/SWC SenderPort  data={'softwarecomponent','AUTOLIV/SoftwareComponents/SAD/SAD','port','pseSolenoidPWM','date',738464.41481978004}  displaystring=SAD\npseSolenoidPWM
  RP_prrFsmProfile : tl_autosar_lib/SWC ReceiverPort  data={'softwarecomponent','AUTOLIV/SoftwareComponents/SAD/SAD','port','prrFsmProfile','date',738430.41689993057}  displaystring=SAD\nprrFsmProfile
  SAD_Init : Subsystem  TreatAsAtomicUnit=on
  SAD_runMainFunction : Subsystem  TreatAsAtomicUnit=on
  SWC ReceiverPort : tl_autosar_lib/SWC ReceiverPort  data={'softwarecomponent','AUTOLIV/SoftwareComponents/SAD/SAD','port','prrSolenoidCurrent','date',738433.42499521992}  displaystring=SAD\nprrSolenoidCurrent
  Terminator : Terminator
  Terminator1 : Terminator
  pseSolenoidPWM : Outport
  wires:
  prrFsmProfile/1 -> RP_prrFsmProfile/1
  RP_prrFsmProfile/1 -> SAD_runMainFunction/1(drparg_au8SelectedProfile)  "au8SelectedProfile"
  sim_au16Current/1 -> SWC ReceiverPort/1
  PP_pseSolenoidPWM/1 -> pseSolenoidPWM/1
  SAD_runMainFunction/1(dsp_au16Pwm) -> PP_pseSolenoidPWM/1  "au16Pwm"
  SAD_Init/1(EN_Boost_1) -> Terminator/1  "pclDioIfServices_WriteChannel"
  SAD_Init/2(EN_Boost_2) -> Terminator1/1
  SWC ReceiverPort/1 -> SAD_runMainFunction/2(sim_au16Current)

== system eCS_Algo_Simulation_2015b_opti - Copy/eCS/Subsystem/eCS/eCS ==
  prrAccelMtrPerSecSqd : Inport
  prrEcsDiagRequest : Inport  Port=2
  BusCreator : BusCreator  Inputs=2
  PP_psrEcsAlgoData : tl_autosar_lib/SWC SenderPort  data={'softwarecomponent','AUTOLIV/SoftwareComponents/eCS/eCS','port','psrEcsAlgoData','date',738573.71918493055}  displaystring=eCS\npsrEcsAlgoData
  RP_prrAccelMtrPerSecSqd : tl_autosar_lib/SWC ReceiverPort  data={'softwarecomponent','AUTOLIV/SoftwareComponents/eCS/eCS','port','prrAccelMtrPerSecSqd','date',738573.71918538189}  displaystring=eCS\nprrAccelMtrPerSecSqd
  RP_prrEcsDiagRequest : tl_autosar_lib/SWC ReceiverPort  data={'softwarecomponent','AUTOLIV/SoftwareComponents/eCS/eCS','port','prrEcsDiagRequest','date',738573.71918555559}  displaystring=eCS\nprrEcsDiagRequest
  eCS_runMainFunction : Subsystem  TreatAsAtomicUnit=on
  psrEcsAlgoData : Outport
  wires:
  prrAccelMtrPerSecSqd/1 -> RP_prrAccelMtrPerSecSqd/1
  prrEcsDiagRequest/1 -> RP_prrEcsDiagRequest/1
  PP_psrEcsAlgoData/1 -> psrEcsAlgoData/1
  BusCreator/1 -> PP_psrEcsAlgoData/1
  RP_prrAccelMtrPerSecSqd/1 -> eCS_runMainFunction/1(drparg_stAccelMtrPerSecSqd)  "stAccelMtrPerSecSqd"
  RP_prrEcsDiagRequest/1 -> eCS_runMainFunction/2(drparg_b8DiagReq)  "b8DiagReq"
  eCS_runMainFunction/1(dsp_b8EcsFlag) -> BusCreator/1  "b8EcsFlag"
  eCS_runMainFunction/2(dsp_u16BallPosition) -> BusCreator/2  "u16BallPosition"

== system eCS_Algo_Simulation_2015b_opti - Copy/FSM/Subsystem/FSM/FSM/FSM_runCheckModeStatus ==
  u32ModesToCheck : Inport  PortDimensions=1  mask(TL_Inport){data={'autosar',{'useautosarcommunication',1,'kind',5,'operationargument','AUTOLIV/SoftwareComponents/FSM/icsModeManagementServices/Operations/CheckModeStatus/OperationArguments/u32ModesToCheck'},'date',738776.6682844907}}
      settings: CopyFcn=if exist('tl_reset_reviewflag') == 2, tl_reset_reviewflag(gcbh); end  DeleteFcn=if exist('delete_tlblock','file')==2,delete_tlblock(gcbh);end  NameChangeFcn=if exist('rename_tlblock','file')==2,rename_tlblock(gcbh);end  OpenFcn=if exist('tl_open_blockdlg','file')==2,tl_open_blockdlg(gcbh);else,open_system(gcbh,'parameter');end
      mask Help: eval(['if exist(''tl_online_help'',''file'') == 2, tl_online_help(''Topic'',''TL_Inport''),else, web([''jar:file:///'',matlabroot,''/help/toolbox/simulink/help.jar!/slref/' lower(get_param(gcbh,'Blocktype')) '.html''], ''-helpbrowser''),end'])
      mask Display: plot([0.2 0.35 NaN 0.65 0.8],[0 1 NaN 0 1]);
  Runnable : tllib/Function  data={'autosar',{'useautosarspecification',1,'softwarecomponent','AUTOLIV/SoftwareComponents/FSM/FSM','runnable','FSM_runCheckModeStatus'},'date',738776.66828332178}  displayString=RUNNABLE
  Src2 : Subsystem
  terminator2 : Terminator
  bModeStatus : Outport  PortDimensions=1  mask(TL_Outport){data={'autosar',{'useautosarcommunication',1,'kind',5,'operationargument','AUTOLIV/SoftwareComponents/FSM/icsModeManagementServices/Operations/CheckModeStatus/OperationArguments/bModeStatus'},'date',738776.66828724532}}
      settings: CopyFcn=if exist('tl_reset_reviewflag') == 2, tl_reset_reviewflag(gcbh); end  DeleteFcn=if exist('delete_tlblock','file')==2,delete_tlblock(gcbh);end  NameChangeFcn=if exist('rename_tlblock','file')==2,rename_tlblock(gcbh);end  OpenFcn=if exist('tl_open_blockdlg','file')==2,tl_open_blockdlg(gcbh);else,open_system(gcbh,'parameter');end
      mask Help: eval(['if exist(''tl_online_help'',''file'') == 2, tl_online_help(''Topic'',''TL_Outport''),else, web([''jar:file:///'',matlabroot,''/help/toolbox/simulink/help.jar!/slref/' lower(get_param(gcbh,'Blocktype')) '.html''], ''-helpbrowser''),end'])
      mask Display: plot([0.2 0.35 NaN 0.65 0.8],[0 1 NaN 0 1]);
  wires:
  u32ModesToCheck/1 -> terminator2/1
  Src2/1(bModeStatus) -> bModeStatus/1

== system eCS_Algo_Simulation_2015b_opti - Copy/FSM/Subsystem/FSM/FSM/FSM_runCheckVehicleInputs ==
  bModeStatus : Inport  PortDimensions=1  mask(TL_Inport){data={'autosar',{'useautosarcommunication',1,'kind',3,'interrunnablevariable','FSM_b8_ModeStatusResult'},'date',738785.60049045144}}
      settings: CopyFcn=if exist('tl_reset_reviewflag','file')==2,tl_reset_reviewflag(gcbh);end  DeleteFcn=if exist('delete_tlblock','file')==2,delete_tlblock(gcbh);end  NameChangeFcn=if exist('rename_tlblock','file')==2,rename_tlblock(gcbh);end  OpenFcn=if exist('tl_open_blockdlg','file')==2,tl_open_blockdlg(gcbh);else,open_system(gcbh,'parameter');end
      mask Help: eval(['if exist(''tl_online_help'',''file'') == 2, tl_online_help(''Topic'',''TL_Inport''),else, web([''jar:file:///'',matlabroot,''/help/toolbox/simulink/help.jar!/slref/' lower(get_param(gcbh,'Blocktype')) '.html''], ''-helpbrowser''),end'])
      mask Display: plot([0.2 0.35 NaN 0.65 0.8],[0 1 NaN 0 1]);
  drparg_u16Vx : Inport  Port=2  PortDimensions=1  mask(TL_Inport){data={'autosar',{'useautosarcommunication',1,'senderreceiverport','prrVehicleInputs','dataelement','u16Vx'},'date',738304.70202324074}}
      settings: CopyFcn=if exist('tl_reset_reviewflag') == 2, tl_reset_reviewflag(gcbh); end  DeleteFcn=if exist('delete_tlblock','file')==2,delete_tlblock(gcbh);end  NameChangeFcn=if exist('rename_tlblock','file')==2,rename_tlblock(gcbh);end  OpenFcn=if exist('tl_open_blockdlg','file')==2,tl_open_blockdlg(gcbh);else,open_system(gcbh,'parameter');end
      mask Help: eval(['if exist(''tl_online_help'',''file'') == 2, tl_online_help(''Topic'',''TL_Inport''),else, web([''jar:file:///'',matlabroot,''/help/toolbox/simulink/help.jar!/slref/' lower(get_param(gcbh,'Blocktype')) '.html''], ''-helpbrowser''),end'])
      mask Display: plot([0.2 0.35 NaN 0.65 0.8],[0 1 NaN 0 1]);
  drparg_u8BuckleState : Inport  Port=3  PortDimensions=1  mask(TL_Inport){data={'autosar',{'useautosarcommunication',1,'senderreceiverport','prrVehicleInputs','dataelement','u8BuckleState'},'date',738304.7020236227}}
      settings: CopyFcn=if exist('tl_reset_reviewflag') == 2, tl_reset_reviewflag(gcbh); end  DeleteFcn=if exist('delete_tlblock','file')==2,delete_tlblock(gcbh);end  NameChangeFcn=if exist('rename_tlblock','file')==2,rename_tlblock(gcbh);end  OpenFcn=if exist('tl_open_blockdlg','file')==2,tl_open_blockdlg(gcbh);else,open_system(gcbh,'parameter');end
      mask Help: eval(['if exist(''tl_online_help'',''file'') == 2, tl_online_help(''Topic'',''TL_Inport''),else, web([''jar:file:///'',matlabroot,''/help/toolbox/simulink/help.jar!/slref/' lower(get_param(gcbh,'Blocktype')) '.html''], ''-helpbrowser''),end'])
      mask Display: plot([0.2 0.35 NaN 0.65 0.8],[0 1 NaN 0 1]);
  For Iterator Subsystem : Subsystem  TreatAsAtomicUnit=on
  Runnable : tllib/Function  data={'autosar',{'useautosarspecification',1,'softwarecomponent','AUTOLIV/SoftwareComponents/FSM/FSM','runnable','FSM_runCheckVehicleInputs'},'date',738304.7020226157}  displayString=RUNNABLE
  ab8IsSolenoidUsed : Outport  PortDimensions=6  mask(TL_Outport){data={'autosar',{'useautosarcommunication',1,'kind',3,'interrunnablevariable','ab8IsSolenoidUsed'},'date',738373.3646115741}}
      settings: CopyFcn=if exist('tl_reset_reviewflag') == 2, tl_reset_reviewflag(gcbh); end  DeleteFcn=if exist('delete_tlblock','file')==2,delete_tlblock(gcbh);end  NameChangeFcn=if exist('rename_tlblock','file')==2,rename_tlblock(gcbh);end  OpenFcn=if exist('tl_open_blockdlg','file')==2,tl_open_blockdlg(gcbh);else,open_system(gcbh,'parameter');end
      mask Help: eval(['if exist(''tl_online_help'',''file'') == 2, tl_online_help(''Topic'',''TL_Outport''),else, web([''jar:file:///'',matlabroot,''/help/toolbox/simulink/help.jar!/slref/' lower(get_param(gcbh,'Blocktype')) '.html''], ''-helpbrowser''),end'])
      mask Display: plot([0.2 0.35 NaN 0.65 0.8],[0 1 NaN 0 1]);
  wires:
  drparg_u16Vx/1 -> For Iterator Subsystem/1(u16Vx)
  drparg_u8BuckleState/1 -> For Iterator Subsystem/2(u8BuckleState)
  For Iterator Subsystem/1(ab8SolenoidEnable) -> ab8IsSolenoidUsed/1
  bModeStatus/1 -> For Iterator Subsystem/3(bModeStatus)
